simulink model "galton_gen_sl"  (Simulink 8.1)
settings: Solver=FixedStepDiscrete  StartTime=0.0  StopTime=10.0  FixedStep=0.1  RelTol=1e-3
settings Model: Creator=zhan  LastModifiedBy=zhan
settings DataIOCC: FinalStateName=XF  SaveFinalState=on  SaveCompleteFinalSimState=on
settings DebuggingCC: StrictBusMsg=Warning
settings SFSimCC: SimParseCustomCode=off

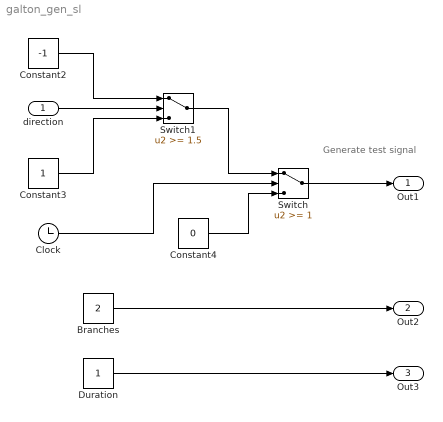
== system galton_gen_sl ==
  note: Generate test signal
  direction : Inport
  Branches : Constant  Value=2
  Clock : Clock
  Constant2 : Constant  Value=-1
  Constant3 : Constant
  Constant4 : Constant  Value=0
  Duration : Constant
  Switch : Switch  Threshold=1
  Switch1 : Switch  Threshold=1.5
  Out1 : Outport
  Out2 : Outport  Port=2
  Out3 : Outport  Port=3
  wires:
  Switch/1 -> Out1/1
  Branches/1 -> Out2/1
  Duration/1 -> Out3/1
  direction/1 -> Switch1/2
  Constant2/1 -> Switch1/1
  Constant3/1 -> Switch1/3
  Clock/1 -> Switch/2
  Switch1/1 -> Switch/1
  Constant4/1 -> Switch/3
